simulink model "dynamic_model_2"  (R2020a)
settings: Solver=FixedStepAuto  StartTime=0.0  StopTime=8*pi  FixedStep=0.05  RelTol=1e-3
libraries: robotmaniplib x1
settings Model: Creator=paolo  LastModifiedBy=paolo

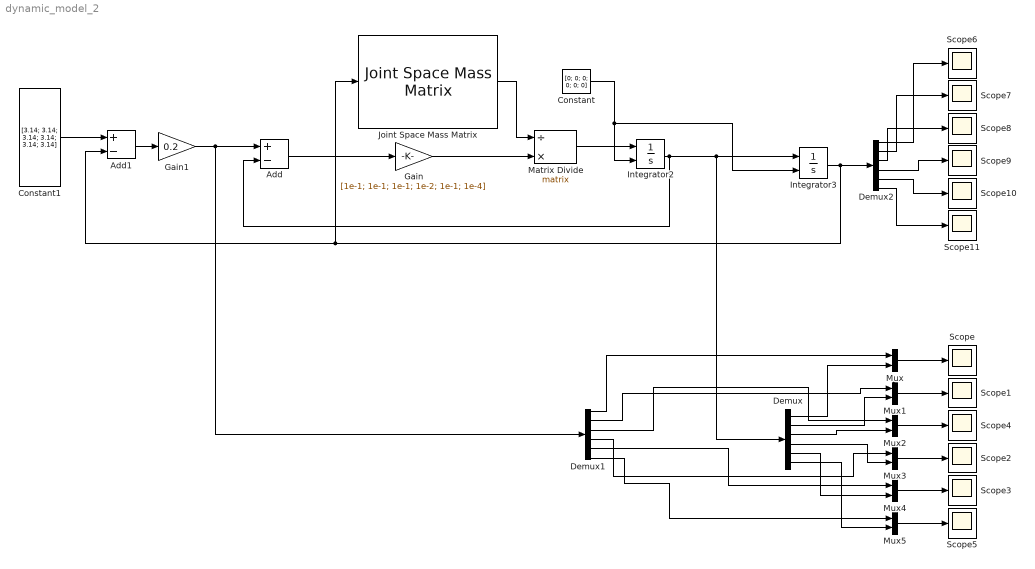
== system dynamic_model_2 ==
  Add : Sum  Inputs=+-
  Add1 : Sum  Inputs=+-
  Constant : Constant  Value=[0; 0; 0; 0; 0; 0]  VectorParams1D=off
  Constant1 : Constant  Value=[3.14; 3.14; 3.14; 3.14; 3.14; 3.14]  VectorParams1D=off
  Demux : Demux  Outputs=6
  Demux1 : Demux  Outputs=6
  Demux2 : Demux  Outputs=6
  Gain : Gain  Gain=[1e-1; 1e-1; 1e-1; 1e-2; 1e-1; 1e-4]
  Gain1 : Gain  Gain=0.2
  Integrator2 : Integrator  InitialConditionSource=external
  Integrator3 : Integrator  InitialConditionSource=external
  Joint Space Mass Matrix : robotmaniplib/Joint Space Mass Matrix  RigidBodyTree=robot  SimulateUsing=Interpreted execution
  Matrix Divide : Product  Inputs=/*  Multiplication=Matrix(*)
  Mux{,1..5} (6 alike) : Mux  Inputs=2
  Scope{,1..11} (12 alike) : Scope
  wires:
  Joint Space Mass Matrix/1 -> Matrix Divide/1
  Constant/1 -> Integrator3/2, Integrator2/2
  Integrator2/1 -> Add/2, Demux/1, Integrator3/1
  Matrix Divide/1 -> Integrator2/1
  Integrator3/1 -> Joint Space Mass Matrix/1, Add1/2, Demux2/1
  Gain1/1 -> Demux1/1, Add/1
  Add/1 -> Gain/1
  Gain/1 -> Matrix Divide/2
  Mux2/1 -> Scope4/1
  Mux1/1 -> Scope1/1
  Mux/1 -> Scope/1
  Mux5/1 -> Scope5/1
  Mux4/1 -> Scope3/1
  Mux3/1 -> Scope2/1
  Demux/6 -> Mux5/2
  Demux/5 -> Mux4/2
  Demux/4 -> Mux3/2
  Demux/3 -> Mux2/2
  Demux/2 -> Mux1/2
  Demux/1 -> Mux/2
  Add1/1 -> Gain1/1
  Constant1/1 -> Add1/1
  Demux1/1 -> Mux/1
  Demux1/2 -> Mux1/1
  Demux1/3 -> Mux2/1
  Demux1/4 -> Mux3/1
  Demux1/5 -> Mux4/1
  Demux1/6 -> Mux5/1
  Demux2/1 -> Scope6/1
  Demux2/2 -> Scope7/1
  Demux2/3 -> Scope8/1
  Demux2/4 -> Scope9/1
  Demux2/5 -> Scope10/1
  Demux2/6 -> Scope11/1
